simulink model "model_walidacyjny_modelu"  (R2020a)
settings: Solver=VariableStepAuto  StartTime=0.0  StopTime=18  RelTol=1e-3
undefined symbols (not defined in the file or in its folder): q0, v0, w0
libraries: powerlib_meascontrol x1
settings Model: Creator=STUDENT  LastModifiedBy=STUDENT

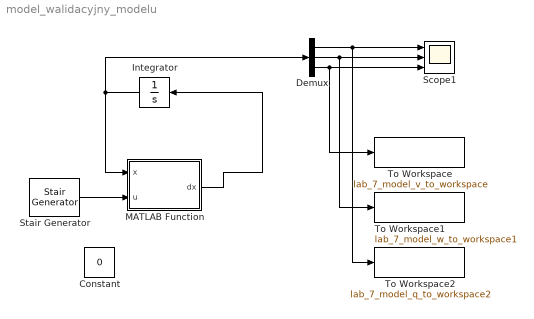
== system model_walidacyjny_modelu ==
  Constant : Constant  Value=0
  Demux : Demux  Outputs=3
  Integrator : Integrator  InitialCondition=[q0, w0, v0]
  MATLAB Function : MATLAB Function  TreatAsAtomicUnit=on
  Scope1 : Scope  NumInputPorts=3
  Stair Generator : powerlib_meascontrol/Pulse & Signal Generators/Stair Generator  t=t_amp_rand2  e=u_amp_rand2_essa  Ts=0.01
  To Workspace : ToWorkspace  VariableName=lab_7_model_v_to_workspace  SaveFormat=Timeseries  SampleTime=0.01
  To Workspace1 : ToWorkspace  VariableName=lab_7_model_w_to_workspace1  SaveFormat=Timeseries  SampleTime=0.01
  To Workspace2 : ToWorkspace  VariableName=lab_7_model_q_to_workspace2  SaveFormat=Timeseries  SampleTime=0.01
  wires:
  MATLAB Function/1(dx) -> Integrator/1
  Integrator/1 -> MATLAB Function/1(x), Demux/1
  Demux/1 -> To Workspace2/1, Scope1/1
  Demux/2 -> To Workspace1/1, Scope1/2
  Demux/3 -> To Workspace/1, Scope1/3
  Stair Generator/1 -> MATLAB Function/2(u)

== matlab function model_walidacyjny_modelu/MATLAB Function ==
  data: x input; u input; dx output
function dx = fcn(x, u)

%dane wyidentyfikowane
% md = 0.0344;
md = 0.028;
g = 9.81;
ksi = 0.01
r = 0.25;
qe = 0.38;
G_estimated = 7287;
J = 0.064675148968382;
% J = 0.1

q = x(1);
w = x(2);
v = x(3);
dx = [0 0 0];
dx(1) = w; % pochodna polozenia
dx(2) = (1/J)*(- md *g * sin(q - qe) - ksi*w - r * Ft(v)); % pochodna predkosci obrotowe belki
dx(3) = G_estimated * (u - uss(v)); %pochodna predkosci smigla 

end


function u = uss(v_d)

    assert(v_d > -3500 && v_d < 3500);
    uss_coef = [1.061404861415565e-11, -8.917411168753438e-10,1.726597501652147e-04,0.001329453668342];
    u = polyval(uss_coef, v_d) ;
    % u = v_d/3500;
    
end 


function sila = Ft(v_2)
    assert(v_2 > -3500 && v_2 < 3500);
    Fc_coef_from_vss = [1.525460520092155e-11,1.434986932293449e-08,6.929547477481372e-05,-0.011003565601160];
    sila = polyval(Fc_coef_from_vss, v_2);
    % sila = v_2/3500*1;
end
